simulink model "Assembly_Quadrotor"  (R2017a)
settings: Solver=ode45  StartTime=0.0  StopTime=30  RelTol=1e-3  EnableMultiTasking=on
undefined symbols (not defined in the file or in its folder): sigbuilder_block, X, Y, Z
libraries: sm_lib x255, nesl_utility x19, simulink x12, fl_lib x4
(part 7 of 7)

== system Assembly_Quadrotor/Quadrotor 3D Model/Quad/MotorD/DCBL_Assembly_CounterClockwise_4_Top_1_RIGID/Assem4DCBL_Assembly_CounterClockwise_4_Top_1_RIGID/hex_nut_style_1_gradeab_iso_1_RIGID ==
  ReferenceFrame : sm_lib/Frames and Transforms/Reference Frame
  Solid : sm_lib/Body Elements/Solid  InertiaType=Custom  Mass=0.00010662444846940384  MassUnits=kg  CenterOfMass=[0 1.3702747535691162e-06 -1.5985959803450969]  CenterOfMassUnits=mm  MomentsOfInertia=[0.00052487586358693401 0.00052487294180577238 0.00087302244809774987]  MomentsOfInertiaUnits=kg*mm^2  ProductsOfInertia=[0 0 0]  ProductsOfInertiaUnits=kg*mm^2  DensityBased=on  Density=1000  DensityUnits=kg/(m^3)  DoExposeReferenceFrame=on  SerializedFrames=<Frames/>  GraphicType=FromGeometry  MarkerShape=Sphere  MarkerSize=10  MarkerSizeUnits=m  GraphicVisPropType=SimpleVisualProperties  GraphicDiffuseColor=[0.77647058823529413 0.75686274509803919 0.73725490196078436]  GraphicSpecularColor=[0.5 0.5 0.5 1.0]  GraphicAmbientColor=[0.15 0.15 0.15 1.0]  GraphicEmissiveColor=[0.0 0.0 0.0 1.0]  GraphicShininess=75  GraphicOpacity=1  GeometryShape=FromFile  RectangleSize=[1 1]  RectangleSizeUnits=m  BrickDimensions=[1 1 1]  BrickDimensionUnits=m  CylinderRadius=1  CylinderRadiusUnits=m  CylinderLength=1  CylinderLengthUnits=m  SphereRadius=1  SphereRadiusUnits=m  EllipsoidRadii=[1 1 1]  EllipsoidRadiiUnits=m  ExtrusionCrossSection=[1 1; -1 1; -1 -1; 1 -1]  ExtrusionCrossSectionUnits=m  ExtrusionLength=1  ExtrusionLengthUnits=m  PolygonNumSides=3  PolygonOuterRadius=1  PolygonOuterRadiusUnits=m  ExtGeomFileType=STL  ExtGeomFileName=hex nut style 1 gradeab_iso_Hexagon Nut ISO - 4032 - M4 - D - N_sldprt.STL  ExtGeomFileUnits=mm  RevolutionCrossSection=[1 1; 1 -1; 2 -1; 2 1]  RevolutionCrossSectionUnits=m  RevolutionExtent=Full  RevolutionAngle=180  RevolutionAngleUnits=deg
  F : PMIOPort  Port=1  Side=Left
  connections:
  F/RConn1 -- ReferenceFrame/RConn1 -- Solid/RConn1

== system Assembly_Quadrotor/Quadrotor 3D Model/Quad/MotorD/DCBL_Assembly_CounterClockwise_4_Top_1_RIGID/Assem4DCBL_Assembly_CounterClockwise_4_Top_1_RIGID/x10x4_7_counterclockwise_propeller_1_RIGID ==
  ReferenceFrame : sm_lib/Frames and Transforms/Reference Frame
  Solid : sm_lib/Body Elements/Solid  InertiaType=Custom  Mass=0.0086221636611543556  MassUnits=kg  CenterOfMass=[5.0000063702530122 5.136767030722547 3.7999863031218535]  CenterOfMassUnits=mm  MomentsOfInertia=[38.086408780943664 39.145966882895458 1.124519086575168]  MomentsOfInertiaUnits=kg*mm^2  ProductsOfInertia=[-1.7703894482553841e-07 5.5344154529569156 1.457353668708178e-07]  ProductsOfInertiaUnits=kg*mm^2  DensityBased=on  Density=1000  DensityUnits=kg/(m^3)  DoExposeReferenceFrame=on  SerializedFrames=<Frames/>  GraphicType=FromGeometry  MarkerShape=Sphere  MarkerSize=10  MarkerSizeUnits=m  GraphicVisPropType=SimpleVisualProperties  GraphicDiffuseColor=[0.75294117647058822 0.75294117647058822 0.75294117647058822]  GraphicSpecularColor=[0.5 0.5 0.5 1.0]  GraphicAmbientColor=[0.15 0.15 0.15 1.0]  GraphicEmissiveColor=[0.0 0.0 0.0 1.0]  GraphicShininess=75  GraphicOpacity=1  GeometryShape=FromFile  RectangleSize=[1 1]  RectangleSizeUnits=m  BrickDimensions=[1 1 1]  BrickDimensionUnits=m  CylinderRadius=1  CylinderRadiusUnits=m  CylinderLength=1  CylinderLengthUnits=m  SphereRadius=1  SphereRadiusUnits=m  EllipsoidRadii=[1 1 1]  EllipsoidRadiiUnits=m  ExtrusionCrossSection=[1 1; -1 1; -1 -1; 1 -1]  ExtrusionCrossSectionUnits=m  ExtrusionLength=1  ExtrusionLengthUnits=m  PolygonNumSides=3  PolygonOuterRadius=1  PolygonOuterRadiusUnits=m  ExtGeomFileType=STL  ExtGeomFileName=10x4.7-counterclockwise-propeller_Default_sldprt.STL  ExtGeomFileUnits=mm  RevolutionCrossSection=[1 1; 1 -1; 2 -1; 2 1]  RevolutionCrossSectionUnits=m  RevolutionExtent=Full  RevolutionAngle=180  RevolutionAngleUnits=deg
  F : PMIOPort  Port=1  Side=Left
  connections:
  F/RConn1 -- ReferenceFrame/RConn1 -- Solid/RConn1

== matlab function Assembly_Quadrotor/Quadrotor 3D Model/Base and Sensor/ConvertAngle1 ==
  data: AngleDeg input; AngleFix output
function AngleFix = getAngleDeg(AngleDeg)
%#codegen
if AngleDeg > 0
    AngleFix = mod(AngleDeg,360);
else
    AngleFix = -mod(abs(AngleDeg),360);
end

== matlab function Assembly_Quadrotor/Quadrotor 3D Model/Base and Sensor/ConvertAngle2 ==
  data: AngleDeg input; AngleFix output
function AngleFix = getAngleDeg(AngleDeg)
%#codegen
if AngleDeg > 0
    AngleFix = mod(AngleDeg,360);
else
    AngleFix = -mod(abs(AngleDeg),360);
end

== matlab function Assembly_Quadrotor/Quadrotor 3D Model/Quad/MotorA/Thrust ==
  data: revSpeed input; Thrust output; revCnst input
function Thrust = generateThrust(revSpeed, revCnst)
% Always give positive thrust (Point up)
Thrust = revCnst * (revSpeed^2);
if (Thrust > 0)
   Thrust = Thrust * (-1);
end

== matlab function Assembly_Quadrotor/Quadrotor 3D Model/Quad/MotorB/Thrust ==
  data: revSpeed input; Thrust output; revCnst input
function Thrust = generateThrust(revSpeed, revCnst)
% Always give positive thrust (Point up)
Thrust = revCnst * (revSpeed^2);
if (Thrust > 0)
   Thrust = Thrust * (-1);
end

== matlab function Assembly_Quadrotor/Quadrotor 3D Model/Quad/MotorC/Thrust ==
  data: revSpeed input; Thrust output; revCnst input
function Thrust = generateThrust(revSpeed, revCnst)
% Always give positive thrust (Point up)
Thrust = revCnst * (revSpeed^2);
if (Thrust > 0)
   Thrust = Thrust * (-1);
end

== matlab function Assembly_Quadrotor/Quadrotor 3D Model/Quad/MotorD/Thrust ==
  data: revSpeed input; Thrust output; revCnst input
function Thrust = generateThrust(revSpeed, revCnst)
% Always give positive thrust (Point up)
Thrust = revCnst * (revSpeed^2);
if (Thrust > 0)
   Thrust = Thrust * (-1);
end

== matlab function Assembly_Quadrotor/Quadrotor 3D Model/Base and Sensor/ConvertAngle ==
  data: AngleDeg input; AngleFix output
function AngleFix = getAngleDeg(AngleDeg)
%#codegen
if AngleDeg > 0
    AngleFix = mod(AngleDeg,360);
else
    AngleFix = -mod(abs(AngleDeg),360);
end
